simulink model "Practica_2_Simulink"  (R2024b)
settings: Solver=VariableStepAuto  StartTime=0.0  StopTime=10  RelTol=1e-3
InitFcn:
  | Ip=0.0079;
  | Mc=0.7031;
  | Lp=0.3302;
  | Mp=0.23;
  | Beq=4.3;
  | g=9.81;
  | Bp=0.0024;
  | Fc=0;
settings Model: Creator=newju  LastModifiedBy=newju

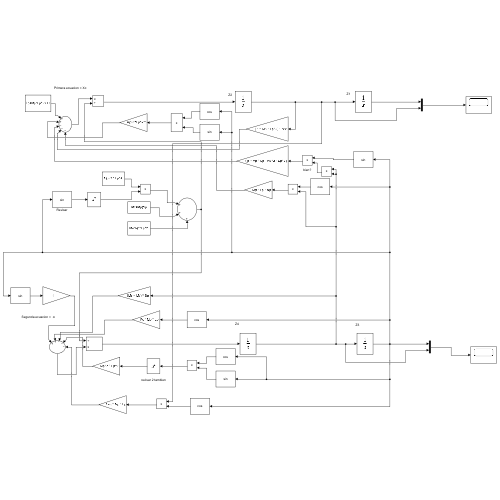
[thumbnail: Simulink's stored preview of the top-level diagram]
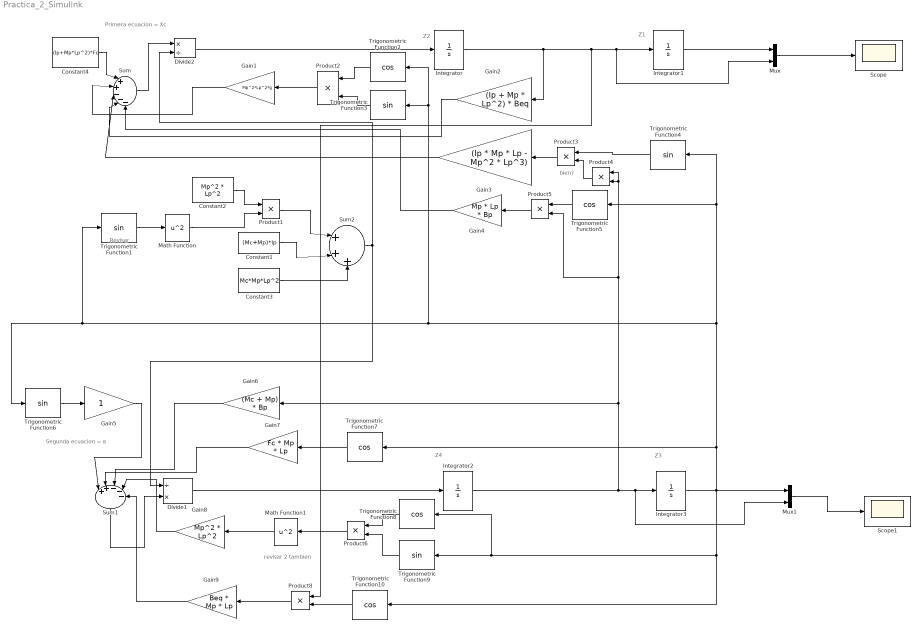
== system Practica_2_Simulink ==
  note: revisar 2 tambien
  note: bien?
  note: Revisar
  note: Z4
  note: Z3
  note: Z1
  note: Z2
  note: Segunda ecuacion = α
  note: Primera ecuacion = Xc
  Constant1 : Constant  Value=(Mc+Mp)*Ip
  Constant2 : Constant  Value=Mp^2 * Lp^2
  Constant3 : Constant  Value=Mc*Mp*Lp^2
  Constant4 : Constant  Value=(Ip+Mp*Lp^2)*Fc
  Divide1 : Product  Inputs=/*
  Divide2 : Product  Inputs=*/
  Gain1 : Gain  Gain=Mp^2*Lp^2*g
  Gain2 : Gain  Gain=(Ip + Mp * Lp^2) * Beq
  Gain3 : Gain  Gain=(Ip * Mp * Lp - Mp^2 * Lp^3)
  Gain4 : Gain  Gain=Mp * Lp * Bp
  Gain5 : Gain
  Gain6 : Gain  Gain=(Mc + Mp) * Bp
  Gain7 : Gain  Gain=Fc * Mp * Lp
  Gain8 : Gain  Gain=Mp^2 * Lp^2
  Gain9 : Gain  Gain=Beq * Mp * Lp
  Integrator : Integrator
  Integrator1 : Integrator
  Integrator2 : Integrator
  Integrator3 : Integrator  InitialCondition=1 * pi/180
  Math Function : Math  Operator=square
  Math Function1 : Math  Operator=square
  Mux : Mux  Inputs=2
  Mux1 : Mux  Inputs=2
  Product{1..6,8} (7 alike) : Product
  Scope : Scope
  Scope1 : Scope
  Sum : Sum  Inputs=|++---
  Sum1 : Sum  Inputs=|++---
  Sum2 : Sum  Inputs=|+++
  Trigonometric Function{1,3..4,6,9} (5 alike) : Trigonometry
  Trigonometric Function{2,5,7..8,10} (5 alike) : Trigonometry  Operator=cos
  wires:
  Mux1/1 -> Scope1/1
  Integrator3/1 -> Trigonometric Function10/1, Trigonometric Function8/1, Trigonometric Function9/1, Trigonometric Function4/1, Trigonometric Function5/1, Trigonometric Function2/1, Trigonometric Function3/1, Trigonometric Function6/1, Trigonometric Function1/1, Trigonometric Function7/1, Mux1/1
  Mux/1 -> Scope/1
  Integrator1/1 -> Mux/1
  Integrator/1 -> Gain2/1, Product8/1, Mux/2, Integrator1/1
  Integrator2/1 -> Gain6/1, Product5/2, Product4/2, Product4/1, Mux1/2, Integrator3/1
  Sum/1 -> Divide2/1
  Constant1/1 -> Sum2/2
  Constant3/1 -> Sum2/3
  Product1/1 -> Sum2/1
  Sum2/1 -> Divide2/2, Divide1/1
  Trigonometric Function1/1 -> Math Function/1
  Divide2/1 -> Integrator/1
  Divide1/1 -> Integrator2/1
  Math Function/1 -> Product1/2
  Constant2/1 -> Product1/1
  Constant4/1 -> Sum/1
  Gain1/1 -> Sum/2
  Trigonometric Function2/1 -> Product2/1
  Trigonometric Function3/1 -> Product2/2
  Product2/1 -> Gain1/1
  Gain2/1 -> Sum/4
  Gain3/1 -> Sum/3
  Product3/1 -> Gain3/1
  Trigonometric Function4/1 -> Product3/1
  Product4/1 -> Product3/2
  Gain4/1 -> Sum/5
  Product5/1 -> Gain4/1
  Trigonometric Function5/1 -> Product5/1
  Sum1/1 -> Divide1/2
  Gain5/1 -> Sum1/1
  Trigonometric Function6/1 -> Gain5/1
  Gain6/1 -> Sum1/3
  Gain7/1 -> Sum1/2
  Trigonometric Function7/1 -> Gain7/1
  Trigonometric Function9/1 -> Product6/2
  Trigonometric Function8/1 -> Product6/1
  Product6/1 -> Math Function1/1
  Math Function1/1 -> Gain8/1
  Gain8/1 -> Sum1/4
  Gain9/1 -> Sum1/5
  Product8/1 -> Gain9/1
  Trigonometric Function10/1 -> Product8/2
